simulink model "LongitudinalModel"  (R2025b)
settings: Solver=VariableStepAuto  StartTime=0.0  StopTime=10  RelTol=1e-3
settings Model: Creator=gonza  LastModifiedBy=gonza

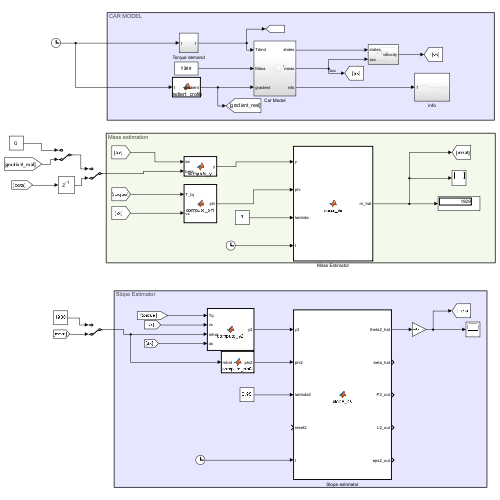
[thumbnail: Simulink's stored preview of the top-level diagram]
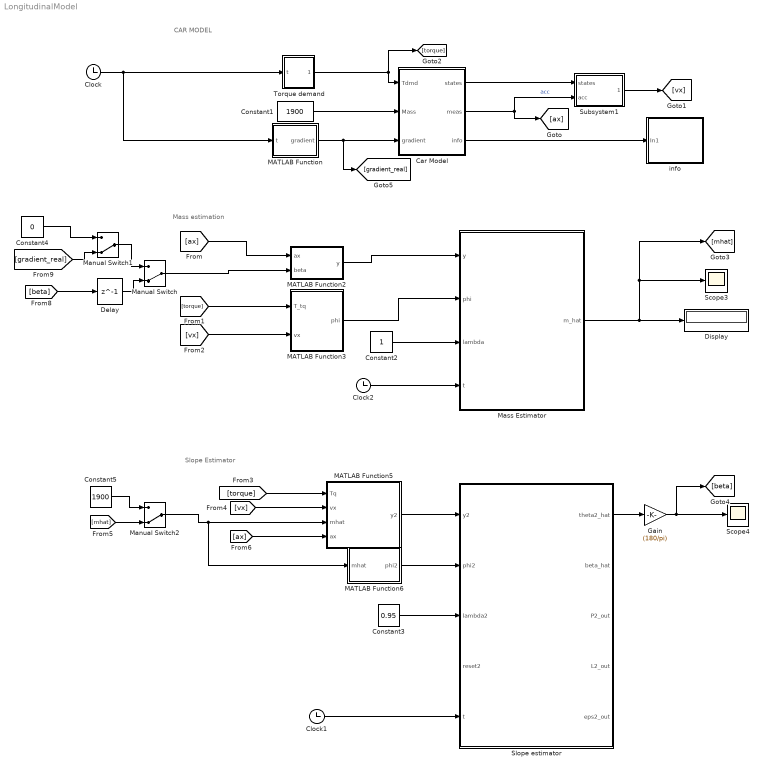
== system LongitudinalModel ==
  note: Slope Estimator
  note: Mass estimation
  note: CAR MODEL
  Car Model : Subsystem
  Clock : Clock
  Clock1 : Clock
  Clock2 : Clock
  Constant1 : Constant  Value=1900
  Constant2 : Constant
  Constant3 : Constant  Value=0.95
  Constant4 : Constant  Value=0
  Constant5 : Constant  Value=1900
  Delay : Delay  DelayLength=1  InputProcessing=Columns as channels (frame based)
  Display : Display
  Gain : Gain  Gain=(180/pi)
  MATLAB Function : MATLAB Function  TreatAsAtomicUnit=on
  MATLAB Function2 : MATLAB Function  TreatAsAtomicUnit=on
  MATLAB Function3 : MATLAB Function  TreatAsAtomicUnit=on
  MATLAB Function5 : MATLAB Function  TreatAsAtomicUnit=on
  MATLAB Function6 : MATLAB Function  TreatAsAtomicUnit=on
  Manual Switch : ManualSwitch  CurrentSetting=0
  Manual Switch1 : ManualSwitch  CurrentSetting=0
  Manual Switch2 : ManualSwitch  CurrentSetting=0
  Mass Estimator : MATLAB Function  TreatAsAtomicUnit=on
  Scope3 : Scope
      settings: ActiveDisplayYMinimum=1650  ActiveDisplayYMaximum=3150  DataLoggingVariableName=ScopeData5
  Scope4 : Scope
      settings: ActiveDisplayYMinimum=-1.3579506202953535  ActiveDisplayYMaximum=12.221555582658183  DataLoggingVariableName=ScopeData6
  Slope estimator : MATLAB Function  TreatAsAtomicUnit=on
  Subsystem1 : Subsystem
  Torque demand : Subsystem
  info : Subsystem
  wires:
  Car Model/3(info) -> info/1(In1)
  Clock/1 -> MATLAB Function/1(t), Torque demand/1(t)
  Constant1/1 -> Car Model/2(Mass)
  Car Model/2(meas) -> [ax], Subsystem1/2(acc)  "acc"
  Subsystem1/1(velocity) -> [vx]
  Car Model/1(states) -> Subsystem1/1(states)
  Torque demand/1(Out1) -> [torque], Car Model/1(Tdmd)
  MATLAB Function/1(gradient) -> [gradient_real], Car Model/3(gradient)
  [torque] -> MATLAB Function3/1(T_tq)
  Constant2/1 -> Mass Estimator/3(lambda)
  [vx] -> MATLAB Function3/2(vx)
  [ax] -> MATLAB Function2/1(ax)
  MATLAB Function2/1(y) -> Mass Estimator/1(y)
  MATLAB Function3/1(phi) -> Mass Estimator/2(phi)
  Manual Switch/1 -> MATLAB Function2/2(beta)
  [torque] -> MATLAB Function5/1(Tq)
  [vx] -> MATLAB Function5/2(vx)
  [ax] -> MATLAB Function5/4(ax)
  MATLAB Function5/1(y2) -> Slope estimator/1(y2)
  MATLAB Function6/1(phi2) -> Slope estimator/2(phi2)
  Constant3/1 -> Slope estimator/3(lambda2)
  Clock1/1 -> Slope estimator/5(t)
  Slope estimator/1(theta2_hat) -> Gain/1
  [beta] -> Delay/1
  Delay/1 -> Manual Switch/2
  Manual Switch1/1 -> Manual Switch/1
  [gradient_real] -> Manual Switch1/2
  Constant4/1 -> Manual Switch1/1
  [mhat] -> Manual Switch2/2
  Constant5/1 -> Manual Switch2/1
  Manual Switch2/1 -> MATLAB Function6/1(mhat), MATLAB Function5/3(mhat)
  Gain/1 -> [beta], Scope4/1
  Mass Estimator/1(m_hat) -> Scope3/1, [mhat], Display/1
  Clock2/1 -> Mass Estimator/4(t)

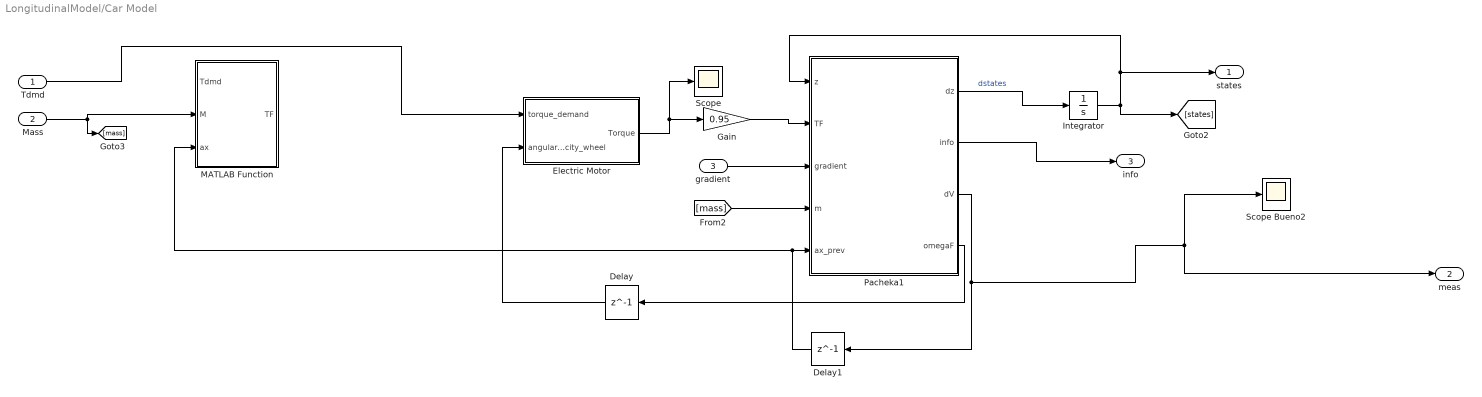
== system LongitudinalModel/Car Model ==
  Tdmd : Inport
  Mass : Inport  Port=2
  gradient : Inport  Port=3
  Delay : Delay  DelayLength=1  InputProcessing=Columns as channels (frame based)  SampleTime=0.01
  Delay1 : Delay  DelayLength=1  InputProcessing=Columns as channels (frame based)  SampleTime=0.01
  Electric Motor : Subsystem
  Gain : Gain  Gain=0.95
  Integrator : Integrator  InitialCondition=[0;0]
  MATLAB Function : MATLAB Function  TreatAsAtomicUnit=on
  Pacheka1 : MATLAB Function  TreatAsAtomicUnit=on
  Scope : Scope
      settings: ActiveDisplayYMinimum=2184.8205164585697  ActiveDisplayYMaximum=2338.8181044267876  DataLoggingVariableName=ScopeData2
  Scope Bueno2 : Scope
      settings: ActiveDisplayYMinimum=-0.33664589083368035  ActiveDisplayYMaximum=1.5583130175031235
  states : Outport
  meas : Outport  Port=2
  info : Outport  Port=3
  wires:
  gradient/1 -> Pacheka1/3(gradient)
  [mass] -> Pacheka1/4(m)
  Pacheka1/1(dz) -> Integrator/1  "dstates"
  Pacheka1/3(dV) -> Delay1/1, meas/1, Scope Bueno2/1
  Pacheka1/4(omegaF) -> Delay/1
  Integrator/1 -> states/1, Pacheka1/1(z), [states]
  Electric Motor/1(Torque) -> Scope/1, Gain/1
  Pacheka1/2(info) -> info/1
  Mass/1 -> [mass], MATLAB Function/2(M)
  Delay1/1 -> Pacheka1/5(ax_prev), MATLAB Function/3(ax)
  Delay/1 -> Electric Motor/2(angular_velocity_wheel)
  Tdmd/1 -> Electric Motor/1(torque_demand)
  Gain/1 -> Pacheka1/2(TF)

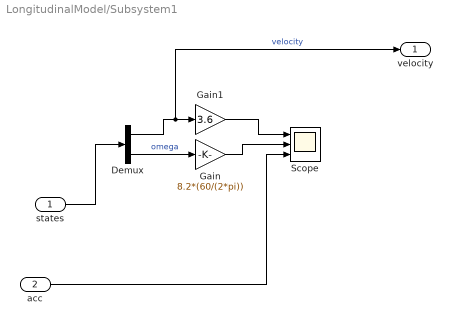
== system LongitudinalModel/Subsystem1 ==
  states : Inport
  acc : Inport  Port=2
  Demux : Demux  Outputs=2
  Gain : Gain  Gain=8.2*(60/(2*pi))
  Gain1 : Gain  Gain=3.6
  Scope : Scope  NumInputPorts=3
      settings: ActiveDisplayYMinimum=-2.6299920402646655  ActiveDisplayYMaximum=23.483796739967332
  velocity : Outport
  wires:
  Gain1/1 -> Scope/1
  Demux/1 -> velocity/1, Gain1/1  "velocity"
  Gain/1 -> Scope/2
  Demux/2 -> Gain/1  "omega"
  states/1 -> Demux/1
  acc/1 -> Scope/3

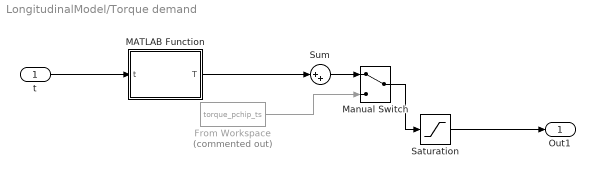
== system LongitudinalModel/Torque demand ==
  t : Inport
  From Workspace : FromWorkspace  Commented=on  VariableName=torque_pchip_ts
  MATLAB Function : MATLAB Function  TreatAsAtomicUnit=on
  Manual Switch : ManualSwitch
  Saturation : Saturate  UpperLimit=2300  LowerLimit=-2300
  Sum : Sum  Inputs=|++
  Out1 : Outport
  wires:
  Saturation/1 -> Out1/1
  From Workspace/1 -> Manual Switch/2
  Manual Switch/1 -> Saturation/1
  Sum/1 -> Manual Switch/1
  MATLAB Function/1(T) -> Sum/1
  t/1 -> MATLAB Function/1(t)
  ? -> Sum/2

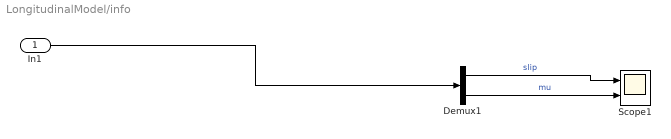
== system LongitudinalModel/info ==
  In1 : Inport
  Demux1 : Demux  Outputs=2
  Scope1 : Scope  NumInputPorts=2
      settings: ActiveDisplayYMinimum=-0.014147564437862976  ActiveDisplayYMaximum=0.064914193473776888  DataLoggingVariableName=ScopeData3
  wires:
  Demux1/2 -> Scope1/2  "mu"
  Demux1/1 -> Scope1/1  "slip"
  In1/1 -> Demux1/1

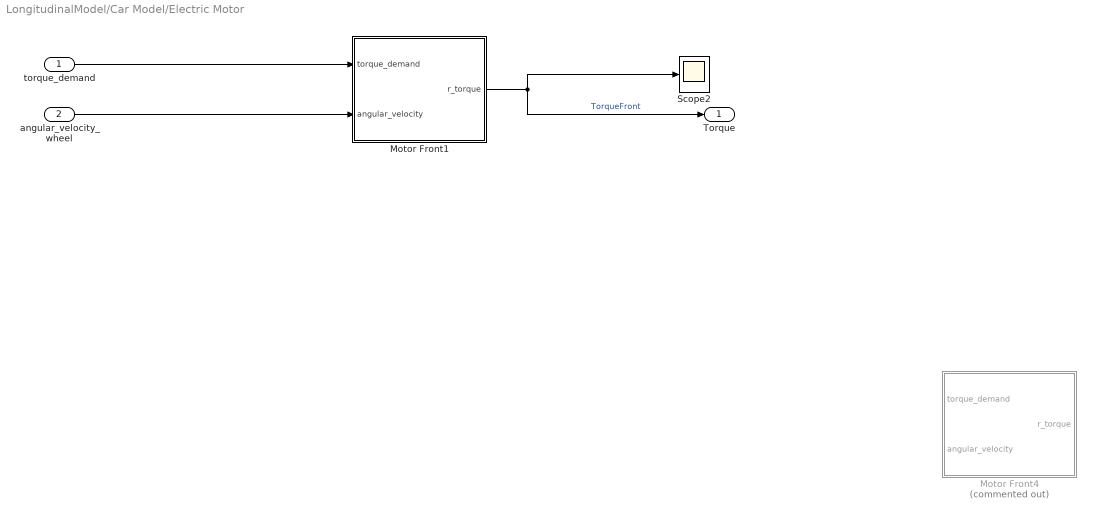
== system LongitudinalModel/Car Model/Electric Motor ==
  torque_demand : Inport
  angular_velocity_wheel : Inport  Port=2
  Motor Front1 : MATLAB Function  TreatAsAtomicUnit=on
  Motor Front4 : MATLAB Function  Commented=on  TreatAsAtomicUnit=on
  Scope2 : Scope
      settings: ActiveDisplayYMinimum=-171.10340073529409  ActiveDisplayYMaximum=1539.9306066176471  DataLoggingVariableName=ScopeData8
  Torque : Outport
  wires:
  angular_velocity_wheel/1 -> Motor Front1/2(angular_velocity)
  Motor Front1/1(r_torque) -> Scope2/1, Torque/1  "TorqueFront"
  torque_demand/1 -> Motor Front1/1(torque_demand)

== matlab function LongitudinalModel/MATLAB Function3 ==
  data: T_tq input; phi output; vx input
function phi = compute_phi(T_tq, vx)

eta=0.95;
re=0.28;

rho = 1.2;
Cd  = 0.29;
A   = 2.4;

F_trac = (T_tq*eta) / re;
F_aero = 0.5 * Cd * A * rho * vx * vx;

phi = F_trac - F_aero;

== matlab function LongitudinalModel/Slope estimator ==
  settings: updateMethod=DISCRETE
  data: y2 input; theta2_hat output; phi2 input; lambda2 input; reset2 input; beta_hat output; P2_out output; L2_out output; eps2_out output; t input
function [theta2_hat, beta_hat, P2_out, L2_out, eps2_out] = slope_rls(y2, phi2, lambda2, reset2, t)

    persistent theta2 P2 initialized2

    if isempty(initialized2) || reset2
        theta2 = 0;    % Initial guess for slope-related parameter
        P2 = 1e6;      % Large initial covariance
        initialized2 = true;
    end

    % Hold estimator during first second
    if t < 5
        theta2_hat = theta2;
        beta_hat   = theta2;
        P2_out     = P2;
        L2_out     = 0;
        eps2_out   = 0;
        return
    end

    % Prediction error
    eps2 = y2 - phi2 * theta2;

    % RLS gain
    L2 = (P2 * phi2) / (lambda2 + phi2 * P2 * phi2);

    % Parameter update
    theta2 = theta2 + L2 * eps2;

    % Covariance update
    P2 = (P2 * (1 - L2 * phi2)) / lambda2;

    % Outputs
    theta2_hat = theta2;
    beta_hat   = theta2_hat;

    P2_out   = P2;
    L2_out   = L2;
    eps2_out = eps2;
end

== matlab function LongitudinalModel/MATLAB Function5 ==
  data: Tq input; y2 output; vx input; mhat input; ax input
function y2 = compute_y2(Tq, vx, mhat,ax)

eta=0.95;
re=0.28;

rho = 1.2;
Cd  = 0.29;
g= 9.81;
A   = 2.4;
f=0.015;
F_aero = 0.5 * Cd * A * rho * vx * vx;
F_rolling = mhat * g * f;

y2 = (Tq)*eta/re -F_aero - F_rolling- mhat * ax;

== matlab function LongitudinalModel/MATLAB Function6 ==
  data: mhat input; phi2 output
function phi2 = compute_phi2(mhat)
g=9.81;

phi2 = mhat * g;

== matlab function LongitudinalModel/MATLAB Function ==
  data: t input; gradient output
function gradient = gradient_profile(t)

grad_final = 10 * pi / 180;   % 5 degrees in radians

t0 = 5;   % start ramp
t1 = 6;   % end ramp

if t < t0
    gradient = 0;

elseif t < t1
    gradient = grad_final * (t - t0) / (t1 - t0);

else
    gradient = grad_final;
end

== matlab function LongitudinalModel/Car Model/Electric Motor/Motor Front1 ==
  data: torque_demand input; angular_velocity input; r_torque output
function r_torque = fcn(torque_demand, angular_velocity)

%#codegen
i = 8.2;
Tmax_drive = 2285/i;
Tmax_regen = 120;     % example
Pmax_drive = 150000;
Pmax_regen = 60000;   % example
i = 8.2;

% Convert wheel -> motor
omega_m = angular_velocity * i;
Tcmd_m  = torque_demand / i;
w = abs(omega_m);

if Tcmd_m >= 0
    % Drive mode
    Tlim = Tmax_drive;
    if w > 1
        Tlim = min(Tlim, Pmax_drive / w);
    end
    Tact_m = min(Tcmd_m, Tlim);
else
    % Regen mode
    Tlim = Tmax_regen;
    if w > 1e-4
        Tlim = min(Tlim, Pmax_regen / w);
    end
    Tact_m = max(Tcmd_m, -Tlim);
end

% Back to wheel
r_torque = Tact_m * i;

end

== matlab function LongitudinalModel/Torque demand/MATLAB Function ==
  data: t input; T output
function T = torque_profile(t)

Tmax1 = 2300;
Tmax2 = 2300;

% First pulse
t0 = 0.01;    
t1 = 2.0;    
t2 = 3.5;    

% Second pulse
t3 = 5.5;    
t4 = 7.0;    
t5 = 8.5;    

% Slopes
slope_up1   = Tmax1 / (t1 - t0);
slope_down1 = -Tmax1 / (t2 - t1);

slope_up2   = Tmax2 / (t4 - t3);
slope_down2 = -Tmax2 / (t5 - t4);

if t < t0
    T = 0;

elseif t < t1
    T = slope_up1 * (t - t0);

elseif t < t2
    T = Tmax1 + slope_down1 * (t - t1);

elseif t < t3
    T = 0;

elseif t < t4
    T = slope_up2 * (t - t3);

elseif t < t5
    T = Tmax2 + slope_down2 * (t - t4);

else
    T = 0;
end

== matlab function LongitudinalModel/Mass Estimator ==
  settings: updateMethod=DISCRETE
  data: y input; phi input; lambda input; m_hat output; t input
function m_hat = mass_rls(y, phi, lambda, t)

    persistent theta P initialized

    if isempty(initialized)
        theta = 1/1800;   % Initial guess for 1/m
        P = 1e6;          % Large initial covariance
        initialized = true;
    end

    theta_min = 1/3000;
    theta_max = 1/1800;

    % Only estimate during first 5 seconds
    if t <= 4
        % Prediction error
        eps = y - phi * theta;

        % RLS gain
        L = (P * phi) / (lambda + phi * P * phi);

        % Parameter update
        theta = theta + L * eps;

        % Covariance update
        P = (P * (1 - L * phi)) / lambda;

        % Saturate theta so that mass stays between 1800 and 3000 kg
        if theta < theta_min
            theta = theta_min;
        elseif theta > theta_max
            theta = theta_max;
        end
    end

    % After 5 s, theta is frozen and m_hat stays constant
    m_hat = 1 / theta;
end

== matlab function LongitudinalModel/MATLAB Function2 ==
  data: ax input; y output; beta input
function y = compute_y(ax,beta) 
g=9.81; 
f=0.015; 
delta=1; 
y = delta*ax + g*f + g*sin(beta);

== matlab function LongitudinalModel/Car Model/Electric Motor/Motor Front4 ==
  data: torque_demand input; angular_velocity input; r_torque output
function r_torque = fcn(torque_demand,angular_velocity)



%#codegen

Tmax_m = 440;     % Nm motor
Pmax   = 220000;     % W  motor
i      = 7;        % gear ratio
epsw   = 1.0;       % rad/s

% convert wheel -> motor
omega_m = angular_velocity * i;
Tcmd_m  = torque_demand / i;

% compute power consistently (motor domain)
power = Tcmd_m * omega_m;

% motor torque limit: constant torque + constant power
Tlim_m = Tmax_m;

w = abs(omega_m);
if w > 0.0001
    TlimP_m = Pmax / w;
    Tlim_m  = min(Tlim_m, TlimP_m);
end

% saturate motor torque (symmetric)
Tact_m = min(max(Tcmd_m, -Tlim_m), Tlim_m);

% back to wheel
r_torque = Tact_m * i;
end

== matlab function LongitudinalModel/Car Model/MATLAB Function ==
  data: Tdmd input; M input; TF output; ax input
function TF = fcn(Tdmd,M,ax)

% constants

g=9.81;
lf=1.214;
L=2.72;
lr=L-lf;
h=0.2;
TF =  (Tdmd)/2;  
fF0 = M*g*lr/((lf+lr));
fR0 = M*g*lf/((lf+lr));
Dfz = M*h/L * ax;
fFz = max(fF0 - Dfz,0);
fRz = max(fR0 + Dfz,0);
TF = Tdmd * fFz/(fFz + fRz);

== matlab function LongitudinalModel/Car Model/Pacheka1 ==
  data: dz output; z input; TF input; gradient input; info output; m input; dV output; ax_prev input; omegaF output
function [dz,info,dV,omegaF] = fcn(z,TF,gradient,m,ax_prev)

% -------- Parameters --------
g  = 9.81;      % m/s^2
Jw = 1.5;       % wheel inertia [kg*m^2
Rw = 0.28;       % wheel radius [m]
Ck=  130000;  %N/m

lf=1.214;
L=2.72;
lr=L-lf;
h=0.4;

rho = 1.2;
Cd  = 0.29;
A   = 2.4;
Crr = 0.015;
% -------- Unpack states --------
Vx     = z(1);
omegaF = z(2);

%% Calculation Normal forces
fF0 = m*g*lr/((lf+lr));
Dfz = m*h/L * ax_prev;
fFz = max(fF0 - Dfz,0);
% -------- Slip calculation --------
epsV=0.1;
denF = max([abs(Vx), abs(omegaF*Rw), epsV]);
sFx  = (omegaF*Rw - Vx) / denF;
% -------- Resistive forces --------
Fdrag = 0.5*rho*Cd*A*Vx^2;
Froll = Crr*m*g;
Fgradient=m*g*sin(gradient);
fFx= Ck*sFx;
mu=fFx/fFz;
%%  Dynamics 
dV      = (fFx - Fdrag - Froll-Fgradient) / m;       % ax_true
domegaF = (TF -fFx*Rw) / Jw;
w_eps = 1.0; % rad/s
if omegaF < w_eps && domegaF < 0
    domegaF = domegaF * (omegaF/w_eps); % se apaga linealmente
end
dz = [dV;domegaF];
ax_prev = dV;
info=[sFx;mu];

end
